simulink model "chap14_14"  (Simulink 8.7)
settings: Solver=ode3  StartTime=0.0  StopTime=0.0  RelTol=1e-3
undefined symbols (not defined in the file): gray, Rec, SDTV
libraries: visionconversions x1, visionanalysis x1, visionsources x1, visiongeotforms x1
settings Model: Creator=Administrator  LastModifiedBy=asus
settings DataIOCC: SignalLoggingSaveFormat=ModelDataLogs
settings OptimizationCC: ExpressionDepthLimit=2147483647
settings DebuggingCC: SolverPrmCheckMsg=warning  FcnCallInpInsideContextMsg=UseLocalSettings  StateNameClashWarn=warning
settings GRTTargetCC: CombineOutputUpdateFcns=off  GRTInterface=on

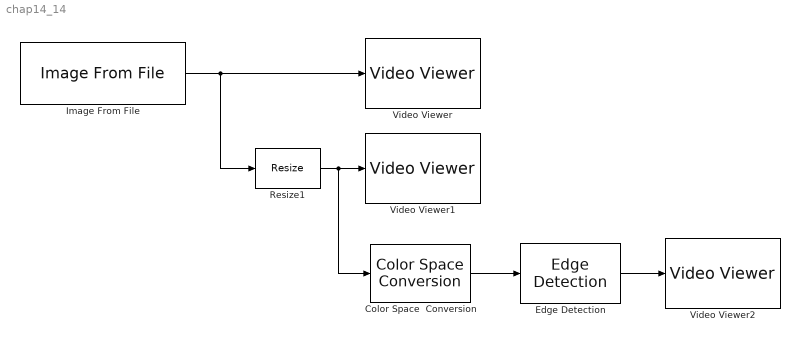
== system chap14_14 ==
  Color Space  Conversion : visionconversions/Color Space  Conversion  conversion=Obsolete  conversionActive=R'G'B' to intensity  wp_str=D65  rec=Rec. 601 (SDTV)  sys=1125/60/2:1  imagePorts=One multidimensional signal
  Edge Detection : visionanalysis/Edge Detection  method=Prewitt  outputType=Binary image  userDefinedThreshold=off  thresholdSource=Input port  threshold=20  thresholdTuning=4  edgeThinning=off  threshold_canny=[0.25 0.60]  autoPercent=70  sigma=1  prodOutputMode=Binary point scaling  prodOutputWordLength=32  prodOutputFracLength=8  roundingMode=Floor  overflowMode=off
  Image From File : visionsources/Image From File  Tag=vipblks_nd  FileName=saturn.png  imagePorts=One multidimensional signal  Ts=inf  ImageDataType=Inherit from input image  Signed=on  WordLength=16  sdImageDataType=uint(8)  FractionLengthMode=User-defined  FractionLength=15  OutPortLabels=R|G|B
  Resize1 : visiongeotforms/Resize  specify=Output size as a percentage of input size  rfactor=[200 150]  outCols=25  outRows=25  outRowsCols=[25 35]  interp_method=Bilinear  antialias=on  useROI=off  roiFlag=off  prodOutputMode=Binary point scaling  prodOutputWordLength=32  prodOutputFracLength=10  roundingMode=Nearest  overflowMode=on
  Video Viewer : VideoViewer  colormapValue=gray(256)  FigPos=[373.8 766 409.6 300]
  Video Viewer1 : VideoViewer  colormapValue=gray(256)  FigPos=[65.8 587.6 410.4 300]
  Video Viewer2 : VideoViewer  colormapValue=gray(256)  FigPos=[757 641.2 409.6 300]
  wires:
  Image From File/1 -> Resize1/1, Video Viewer/1
  Color Space  Conversion/1 -> Edge Detection/1
  Edge Detection/1 -> Video Viewer2/1
  Resize1/1 -> Color Space  Conversion/1, Video Viewer1/1
